simulink model "Plant"  (R2020b)
settings: Solver=VariableStepAuto  StartTime=0.0  StopTime=10.0  RelTol=1e-3
undefined symbols (not defined in the file): plant_Backlash, plant_Kb, plant_Kk, plant_Kt, plant_Kv, plant_L, plant_R, ts_control
libraries: fl_lib x19, nesl_utility x6, sdl_lib x1
settings Model: DataDictionary=Dictionary.sldd  EnableAccessToBaseWorkspace=off  OrderedModelArguments=off  Creator=elbit  LastModifiedBy=alons

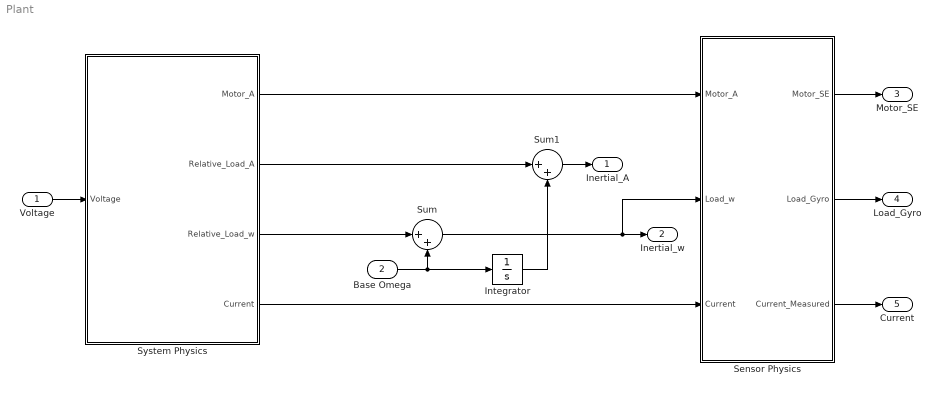
== system Plant ==
  Voltage : Inport  OutDataTypeStr=double  SampleTime=0
  Base Omega : Inport  Port=2  OutDataTypeStr=double  SampleTime=0
  Integrator : Integrator
  Sensor Physics : Subsystem
  Sum : Sum  Inputs=|++
  Sum1 : Sum  Inputs=|++
  System Physics : Subsystem
  Inertial_A : Outport
  Inertial_w : Outport  Port=2
  Motor_SE : Outport  Port=3
  Load_Gyro : Outport  Port=4
  Current : Outport  Port=5
  wires:
  Sensor Physics/1(Motor_SE) -> Motor_SE/1
  Voltage/1 -> System Physics/1(Voltage)
  System Physics/1(Motor_A) -> Sensor Physics/1(Motor_A)
  Sensor Physics/2(Load_Gyro) -> Load_Gyro/1
  System Physics/3(Relative_Load_w) -> Sum/1
  Sum/1 -> Inertial_w/1, Sensor Physics/2(Load_w)
  System Physics/2(Relative_Load_A) -> Sum1/1
  Sum1/1 -> Inertial_A/1
  System Physics/4(Current) -> Sensor Physics/3(Current)
  Sensor Physics/3(Current_Measured) -> Current/1
  Base Omega/1 -> Integrator/1, Sum/2
  Integrator/1 -> Sum1/2

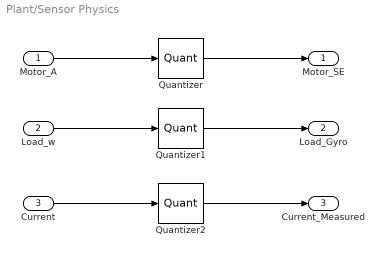
== system Plant/Sensor Physics ==
  Motor_A : Inport
  Load_w : Inport  Port=2
  Current : Inport  Port=3
  Quantizer : Quantizer  QuantizationInterval=2*pi/(2^25)
  Quantizer1 : Quantizer  QuantizationInterval=2*pi/(2^25)/(ts_control)
  Quantizer2 : Quantizer  QuantizationInterval=1e-10
  Motor_SE : Outport
  Load_Gyro : Outport  Port=2
  Current_Measured : Outport  Port=3
  wires:
  Motor_A/1 -> Quantizer/1
  Load_w/1 -> Quantizer1/1
  Quantizer/1 -> Motor_SE/1
  Quantizer1/1 -> Load_Gyro/1
  Quantizer2/1 -> Current_Measured/1
  Current/1 -> Quantizer2/1

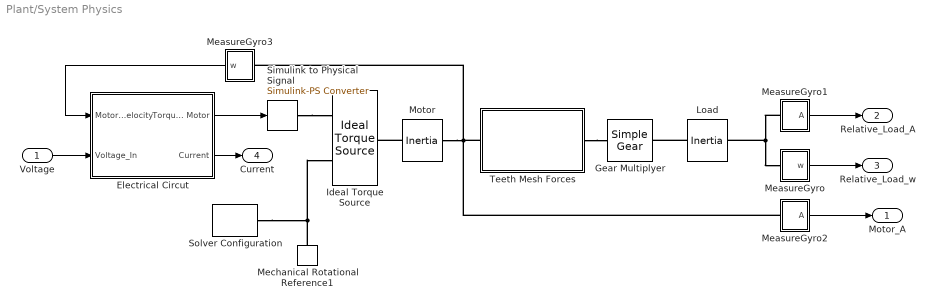
== system Plant/System Physics ==
  Voltage : Inport
  Electrical Circut : Subsystem  mask{K_T=plant_Kt, K_b=plant_Kb, R=plant_R, L=plant_L}
      mask prompts: K_T "K_T [Nm/A]"; K_b "K_b[Vpeak/(rad/s)]"; R "R [Ohm]"; L "L [H]"
      mask init:
      | set_param(gcbh,'backgroundcolor','brown' );
      mask Display:
      | x=0.05+[ 0.4781
      |     0.2730
      |     0.4435
      |     0.2984
      |     0.4412
      |     0.3514
      |     0.5910
      |     0.4435
      |     0.5818
      |     0.4182
      |     0.4781];
      | 
      | y=[ 0.9111
      |     0.5875
      |     0.5816
      |     0.3192
      |     0.3338
      |     0.0423
      |     0.4009
      |     0.4009
      |     0.6516
      |     0.6516
      |     0.9082];
      | 
      | patch(x,y,[0.8,0.7,0.1])
      | plot(x,y)
  Gear Multiplyer : sdl_lib/Gears/Simple Gear  ratio=plant_N  rotation_direction=sdl.enum.shaftOutputDirection.same  friction_model=sdl.enum.gear_efficiencies_load.off  mu_visc=[0, 0] N*m/(rad/s)  T_noload=0.1 N*m  T_nom=5 N*m  efficiency_nom=0.8  efficiency=0.8  temperature_TLU=[280, 300, 320] K  load_TLU=[1, 5, 10] N*m  efficiency_TLU=[.95, .9, .85]  efficiency_TLU2=[.85, .8, .75; .95, .9, .85; .85, .8, .7]  w_thr=0.01 rad/s  pwr_thr=0.001 W  thermal_mass=50 J/K  enable_faults=simscape.enum.onoff.off  efficiency_fault=0.05  external_fault=simscape.enum.onoff.off  temporal_fault=simscape.enum.onoff.off  fault_time=5 s  fault_angles=pi / 12 rad  report_fault=simscape.enum.assert.action.none  temperature_specify=off  temperature_priority=High  temperature=300 K  temperature_nominal_specify=off  temperature_nominal_unit=K  temperature_nominal_value=1
  Ideal Torque Source : fl_lib/Mechanical/Mechanical Sources/Ideal Torque Source
  Load : fl_lib/Mechanical/Rotational Elements/Inertia  inertia=plant_Jload kg*m^2  num_ports=foundation.enum.numPorts2.two  w_specify=off  w_priority=High  w=0 rad/s  w_nominal_specify=off  w_nominal_unit=rad/s  w_nominal_value=1  t_specify=off  t_priority=None  t=0 N*m  t_nominal_specify=off  t_nominal_unit=N*m  t_nominal_value=1
      settings: InternalSimscapePortConfiguration="{\"Bottom\":[],\"Left\":[{\"id\":\"I\",\"label\":\"\",\"type\":\"foundation.mechanical.rotational.rotational\"}],\"Right\":[{\"id\":\"J\",\"label\":\"\",\"type\":\"foundation.mechanical.rotational.rotational\"}],\"Top\":[]}"
  MeasureGyro : Subsystem
      mask Display: disp('w')
  MeasureGyro1 : Subsystem
      mask Display: disp('A')
  MeasureGyro2 : Subsystem
      mask Display: disp('A')
  MeasureGyro3 : Subsystem
      mask Display: disp('w')
  Mechanical Rotational Reference1 : fl_lib/Mechanical/Rotational Elements/Mechanical Rotational Reference
  Motor : fl_lib/Mechanical/Rotational Elements/Inertia  inertia=plant_Jmotor kg*m^2  num_ports=foundation.enum.numPorts2.two  w_specify=off  w_priority=High  w=0 rad/s  w_nominal_specify=off  w_nominal_unit=rad/s  w_nominal_value=1  t_specify=off  t_priority=None  t=0 N*m  t_nominal_specify=off  t_nominal_unit=N*m  t_nominal_value=1
      settings: InternalSimscapePortConfiguration="{\"Bottom\":[],\"Left\":[{\"id\":\"I\",\"label\":\"\",\"type\":\"foundation.mechanical.rotational.rotational\"}],\"Right\":[{\"id\":\"J\",\"label\":\"\",\"type\":\"foundation.mechanical.rotational.rotational\"}],\"Top\":[]}"
  Simulink to Physical Signal : nesl_utility/Simulink-PS Converter  PhysicalDomain=network_engine_domain  SubClassName=ps_input  LeftPortType=input  RightPortType=output  PseudoPeriodic=off  Frequencies=[]  NoiseDistribution=none  NoiseParameters=[]  Unit=N*m  AffineConversion=off  FilteringAndDerivatives=zero  SimscapeFilterOrder=1  InputFilterTimeConstant=.001  UdotUserProvided=0
  Solver Configuration : nesl_utility/Solver Configuration  PhysicalDomain=network_engine_domain  SubClassName=solver  LeftPortType=input  RightPortType=generic  Tones=[]  Harmonics=[]  SimulateNoise=off  Profile=off  UseLocalSampling=off  EnableSwitchedLinearOptims=on  FrequencyDomain=off  UseCCode=off  RelTol=0.001  AbsTol=1e-06  MinStep=1e-09  ToWorkspace=off  RevertToSquareIcSolve=off  NumHomotopyIterations=100  PhasorMode=off  PhasorModeNumHarmonics=1  DoDC=off  ResidualTolerance=1e-09  UseLocalSolver=off  LocalSolverChoice=NE_BACKWARD_EULER_ADVANCER  LocalSolverSampleTime=0.001  DoFixedCost=off  MaxNonlinIter=3  MaxModeIter=2  ComputeImpulses=off  ImpulseIterations=2  LinearAlgebra=auto  EquationFormulation=NE_TIME_EF  DelaysMemoryBudget=1024  AutomaticFiltering=on  FilteringTimeConstant=0.001  PartitionStorageMethod=AS_NEEDED  PartitionMemoryBudget=1024  PartitionMethod=ROBUST
  Teeth Mesh Forces : Subsystem  Variant=on  VariantControlMode=label  VariantControl=Choice  LabelModeActiveChoice=Linear  mask{Kk=plant_Kk, Kv=plant_Kv, Backlash=plant_Backlash}
      mask prompts: Kk "Kk [Nm/rad]"; Kv "Kv [Nm/rad/s]"; Backlash "Backlash [rad]"
  Motor_A : Outport
  Relative_Load_A : Outport  Port=2
  Relative_Load_w : Outport  Port=3
  Current : Outport  Port=4
  wires:
  MeasureGyro1/1(A) -> Relative_Load_A/1
  MeasureGyro/1(w) -> Relative_Load_w/1
  MeasureGyro2/1(A) -> Motor_A/1
  Voltage/1 -> Electrical Circut/2(Voltage_In)
  Electrical Circut/2(Current) -> Current/1
  MeasureGyro3/1(w) -> Electrical Circut/1(Motor Velocity)
  Electrical Circut/1(Torque on Motor) -> Simulink to Physical Signal/1
  connections:
  Load/RConn1 -- MeasureGyro/LConn1 -- MeasureGyro1/LConn1
  Load/LConn1 -- Gear Multiplyer/RConn1
  Motor/LConn1 -- Ideal Torque Source/LConn1
  Teeth Mesh Forces/RConn1 -- Gear Multiplyer/LConn1
  Mechanical Rotational Reference1/LConn1 -- Ideal Torque Source/RConn2 -- Solver Configuration/RConn1
  Simulink to Physical Signal/RConn1 -- Ideal Torque Source/RConn1
  Motor/RConn1 -- Teeth Mesh Forces/LConn1 -- MeasureGyro2/LConn1 -- MeasureGyro3/LConn1

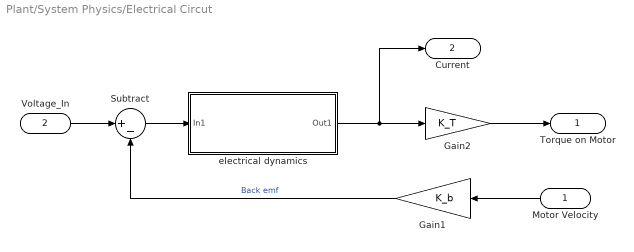
== system Plant/System Physics/Electrical Circut ==
  Motor Velocity : Inport
  Voltage_In : Inport  Port=2
  Gain1 : Gain  Gain=K_b
  Gain2 : Gain  Gain=K_T
  Subtract : Sum  Inputs=|+-
  electrical dynamics : Subsystem
      mask Display: disp('1\n----------\nLs+R')
  Torque on Motor : Outport
  Current : Outport  Port=2
  wires:
  Gain2/1 -> Torque on Motor/1
  Voltage_In/1 -> Subtract/1
  Gain1/1 -> Subtract/2  "Back emf"
  Subtract/1 -> electrical dynamics/1(In1)
  electrical dynamics/1(Out1) -> Current/1, Gain2/1
  Motor Velocity/1 -> Gain1/1

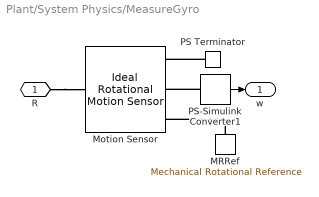
== system Plant/System Physics/MeasureGyro ==
  MRRef : fl_lib/Mechanical/Rotational Elements/Mechanical Rotational Reference
      settings: SourceProductName=Foundation Library
  Motion Sensor : fl_lib/Mechanical/Mechanical Sensors/Ideal Rotational Motion Sensor  wrap_angle=simscape.enum.onoff.off  offset=0 rad
      settings: SourceProductName=Foundation Library
  PS Terminator : fl_lib/Physical Signals/Sinks/PS Terminator
  PS-Simulink Converter1 : nesl_utility/PS-Simulink Converter  PhysicalDomain=network_engine_domain  SubClassName=ps_output  LeftPortType=input  RightPortType=output  PseudoPeriodic=off  Frequencies=[]  Unit=inherit  AffineConversion=off
      settings: SourceProductName=Utilities
  R : PMIOPort  Side=Left
  w : Outport  VectorParamsAs1DForOutWhenUnconnected=off
  wires:
  PS-Simulink Converter1/1 -> w/1
  connections:
  MRRef/LConn1 -- Motion Sensor/RConn1
  R/RConn1 -- Motion Sensor/LConn1
  PS Terminator/LConn1 -- Motion Sensor/RConn3
  PS-Simulink Converter1/LConn1 -- Motion Sensor/RConn2

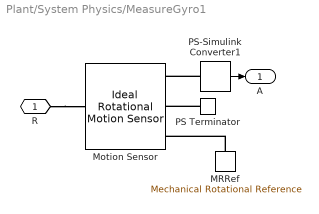
== system Plant/System Physics/MeasureGyro1 ==
  MRRef : fl_lib/Mechanical/Rotational Elements/Mechanical Rotational Reference
      settings: SourceProductName=Foundation Library
  Motion Sensor : fl_lib/Mechanical/Mechanical Sensors/Ideal Rotational Motion Sensor  wrap_angle=simscape.enum.onoff.off  offset=0 rad
      settings: SourceProductName=Foundation Library
  PS Terminator : fl_lib/Physical Signals/Sinks/PS Terminator
  PS-Simulink Converter1 : nesl_utility/PS-Simulink Converter  PhysicalDomain=network_engine_domain  SubClassName=ps_output  LeftPortType=input  RightPortType=output  PseudoPeriodic=off  Frequencies=[]  Unit=inherit  AffineConversion=off
      settings: SourceProductName=Utilities
  R : PMIOPort  Side=Left
  A : Outport  VectorParamsAs1DForOutWhenUnconnected=off
  wires:
  PS-Simulink Converter1/1 -> A/1
  connections:
  MRRef/LConn1 -- Motion Sensor/RConn1
  R/RConn1 -- Motion Sensor/LConn1
  PS-Simulink Converter1/LConn1 -- Motion Sensor/RConn3
  PS Terminator/LConn1 -- Motion Sensor/RConn2

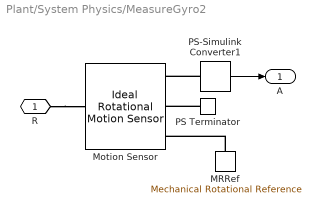
== system Plant/System Physics/MeasureGyro2 ==
  MRRef : fl_lib/Mechanical/Rotational Elements/Mechanical Rotational Reference
      settings: SourceProductName=Foundation Library
  Motion Sensor : fl_lib/Mechanical/Mechanical Sensors/Ideal Rotational Motion Sensor  wrap_angle=simscape.enum.onoff.off  offset=0 rad
      settings: SourceProductName=Foundation Library
  PS Terminator : fl_lib/Physical Signals/Sinks/PS Terminator
  PS-Simulink Converter1 : nesl_utility/PS-Simulink Converter  PhysicalDomain=network_engine_domain  SubClassName=ps_output  LeftPortType=input  RightPortType=output  PseudoPeriodic=off  Frequencies=[]  Unit=inherit  AffineConversion=off
      settings: SourceProductName=Utilities
  R : PMIOPort  Side=Left
  A : Outport  VectorParamsAs1DForOutWhenUnconnected=off
  wires:
  PS-Simulink Converter1/1 -> A/1
  connections:
  MRRef/LConn1 -- Motion Sensor/RConn1
  R/RConn1 -- Motion Sensor/LConn1
  PS-Simulink Converter1/LConn1 -- Motion Sensor/RConn3
  PS Terminator/LConn1 -- Motion Sensor/RConn2

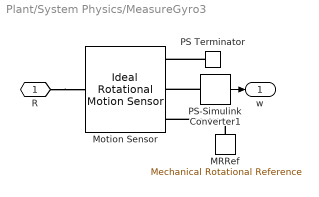
== system Plant/System Physics/MeasureGyro3 ==
  MRRef : fl_lib/Mechanical/Rotational Elements/Mechanical Rotational Reference
      settings: SourceProductName=Foundation Library
  Motion Sensor : fl_lib/Mechanical/Mechanical Sensors/Ideal Rotational Motion Sensor  wrap_angle=simscape.enum.onoff.off  offset=0 rad
      settings: SourceProductName=Foundation Library
  PS Terminator : fl_lib/Physical Signals/Sinks/PS Terminator
  PS-Simulink Converter1 : nesl_utility/PS-Simulink Converter  PhysicalDomain=network_engine_domain  SubClassName=ps_output  LeftPortType=input  RightPortType=output  PseudoPeriodic=off  Frequencies=[]  Unit=inherit  AffineConversion=off
      settings: SourceProductName=Utilities
  R : PMIOPort  Side=Left
  w : Outport  VectorParamsAs1DForOutWhenUnconnected=off
  wires:
  PS-Simulink Converter1/1 -> w/1
  connections:
  MRRef/LConn1 -- Motion Sensor/RConn1
  R/RConn1 -- Motion Sensor/LConn1
  PS Terminator/LConn1 -- Motion Sensor/RConn3
  PS-Simulink Converter1/LConn1 -- Motion Sensor/RConn2

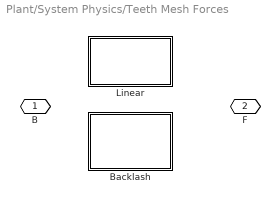
== system Plant/System Physics/Teeth Mesh Forces ==
  Backlash : Subsystem  VariantControl=NonLinear
  Linear : Subsystem  VariantControl=Linear
  B : PMIOPort  Side=Left
  F : PMIOPort  Port=2  Side=Right

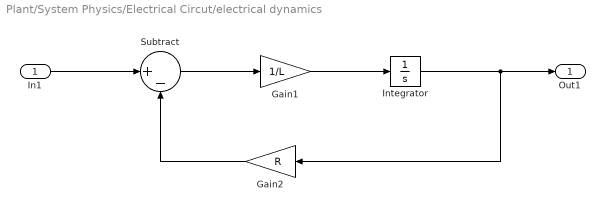
== system Plant/System Physics/Electrical Circut/electrical dynamics ==
  In1 : Inport
  Gain1 : Gain  Gain=1/L
  Gain2 : Gain  Gain=R
  Integrator : Integrator
  Subtract : Sum  Inputs=|+-
  Out1 : Outport
  wires:
  In1/1 -> Subtract/1
  Gain1/1 -> Integrator/1
  Subtract/1 -> Gain1/1
  Gain2/1 -> Subtract/2
  Integrator/1 -> Gain2/1, Out1/1

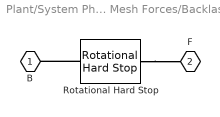
== system Plant/System Physics/Teeth Mesh Forces/Backlash ==
  Rotational Hard Stop : fl_lib/Mechanical/Rotational Elements/Rotational Hard Stop  upper_bnd=Backlash/2 rad  lower_bnd=-Backlash/2 rad  stiff_up=Kk N*m/rad  stiff_low=Kk N*m/rad  D_up=Kv N*m/(rad/s)  D_low=Kv N*m/(rad/s)  model=simscape.enum.hardstop.fulldamped  transition=0.001 rad  w_specify=off  w_priority=None  w=0 rad/s  w_nominal_specify=off  w_nominal_unit=rad/s  w_nominal_value=1  t_specify=off  t_priority=None  t=0 N*m  t_nominal_specify=off  t_nominal_unit=N*m  t_nominal_value=1  phi_specify=off  phi_priority=High  phi=0 rad  phi_nominal_specify=off  phi_nominal_unit=rad  phi_nominal_value=1
      settings: SourceProductBaseCode=SS
  B : PMIOPort  Side=Left
  F : PMIOPort  Port=2  Side=Right
  connections:
  Rotational Hard Stop/RConn1 -- F/RConn1
  Rotational Hard Stop/LConn1 -- B/RConn1

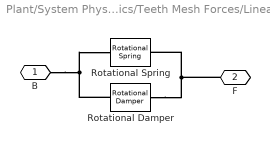
== system Plant/System Physics/Teeth Mesh Forces/Linear ==
  Rotational Damper : fl_lib/Mechanical/Rotational Elements/Rotational Damper  D=Kv N*m/(rad/s)  w_specify=off  w_priority=None  w=0 rad/s  w_nominal_specify=off  w_nominal_unit=rad/s  w_nominal_value=1  t_specify=off  t_priority=None  t=0 N*m  t_nominal_specify=off  t_nominal_unit=N*m  t_nominal_value=1
  Rotational Spring : fl_lib/Mechanical/Rotational Elements/Rotational Spring  spr_rate=Kk N*m/rad  w_specify=off  w_priority=None  w=0 rad/s  w_nominal_specify=off  w_nominal_unit=rad/s  w_nominal_value=1  t_specify=off  t_priority=None  t=0 N*m  t_nominal_specify=off  t_nominal_unit=N*m  t_nominal_value=1  phi_specify=off  phi_priority=High  phi=0 rad  phi_nominal_specify=off  phi_nominal_unit=rad  phi_nominal_value=1
  B : PMIOPort  Side=Left
  F : PMIOPort  Port=2  Side=Right
  connections:
  Rotational Damper/RConn1 -- F/RConn1 -- Rotational Spring/RConn1
  Rotational Damper/LConn1 -- B/RConn1 -- Rotational Spring/LConn1
